simulink model "example_Hydraulic_Valve"  (R2016b)
settings: Solver=ode45  StartTime=0.0  StopTime=210  RelTol=1e-3  EnableMultiTasking=on
libraries: carnot x4, simulink x1
settings Model: Creator=drhf  LastModifiedBy=drhf
settings DataIOCC: LimitDataPoints=on  SaveFormat=Array
settings OptimizationCC: ExpressionDepthLimit=2147483647  LifeSpan=inf
settings DebuggingCC: UnderspecifiedInitializationDetection=Classic  MergeDetectMultiDrivingBlocksExec=none  SolverPrmCheckMsg=warning  StateNameClashWarn=warning  SFUnexpectedBacktrackingDiag=warning  SFNoUnconditionalDefaultTransitionDiag=warning  SFExecutionAtInitializationDiag=none
settings HardwareCC: ProdBitPerPointer=32  ProdBitPerSizeT=32  ProdBitPerPtrDiffT=32  ProdLargestAtomicFloat=None  ProdIntDivRoundTo=Undefined  ProdEndianess=Unspecified  ProdWordSize=32  ProdHWDeviceType=32-bit Generic
settings ModelReferenceCC: PropagateSignalLabelsOutOfModel=off
settings GRTTargetCC: TargetLangStandard=C89/C90 (ANSI)  GeneratePreprocessorConditionals=Disable all  CombineOutputUpdateFcns=off  GRTInterface=on
settings ConfigComp: CovMetricSettings=dw  CovHtmlReporting=on  CovSaveCumulativeToWorkspaceVar=on  CovSaveSingleToWorkspaceVar=on  CovExternalEMLEnable=off

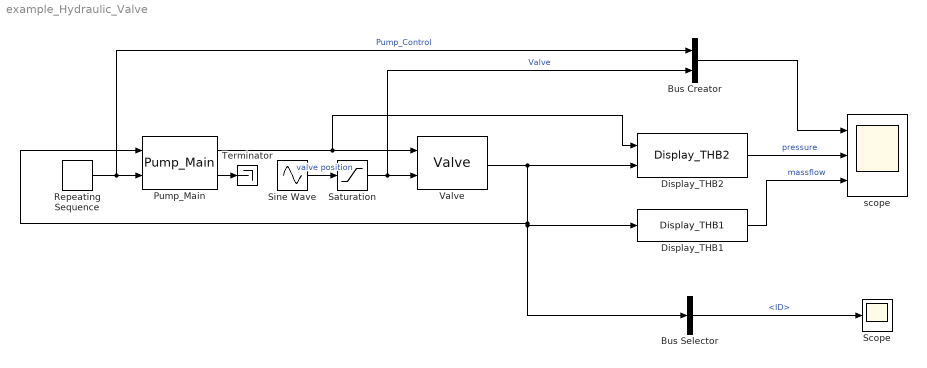
== system example_Hydraulic_Valve ==
  Bus Creator : BusCreator  Inputs=2
  Bus Selector : BusSelector  OutputSignals=ID
  Display_THB1 : carnot/Outputs/Display_THB1  t=off  m=on  p=off  id=off  mix=off  d=off
  Display_THB2 : carnot/Outputs/Display_THB2  t=off  m=off  p=on  id=off  mix=off  d=off
  Pump_Main : carnot/Hydraulics/Pump_Main  a0=2.7e4  a1=-1.2e4  a2=0%-3e-3  dia=0.025  t1=1  p0=3e5  IDchk=off  fluid_id=Water  mix=0  ua=1  mcp=500  tamb=20
  Repeating Sequence : simulink/Sources/Repeating Sequence  rep_seq_t=[0 20 60 200]  rep_seq_y=[0 0 1 1]
  Saturation : Saturate  UpperLimit=1  LowerLimit=0
  Scope : Scope
  Sine Wave : Sin  Amplitude=0.6  Bias=0.5  Frequency=1/20  SampleTime=0
  Terminator : Terminator
  Valve : carnot/Hydraulics/Valve  pos_values=[0 0.1 1]  dp_values=[1e6 1e6 1]
  scope : Scope  NumInputPorts=3
  wires:
  Repeating Sequence/1 -> Bus Creator/1, Pump_Main/2  "Pump_Control"
  Pump_Main/2 -> Terminator/1
  Sine Wave/1 -> Saturation/1  "valve position"
  Pump_Main/1 -> Valve/1, Display_THB2/1
  Display_THB2/1 -> scope/2  "pressure"
  Valve/1 -> Bus Selector/1, Display_THB1/1, Pump_Main/1, Display_THB2/2
  Display_THB1/1 -> scope/3  "massflow"
  Bus Selector/1 -> Scope/1  "<ID>"
  Saturation/1 -> Bus Creator/2, Valve/2  "Valve"
  Bus Creator/1 -> scope/1
